simulink model "System_Design_Quadrocopter"  (Simulink 7.5)
settings: Solver=ode45  StartTime=0.0  StopTime=30  RelTol=1e-3
values from neighbouring files (symbols this model uses):
  phi0 = 0.15    [Quadrocopter_control_Driver.m]    (also in calc_stability.m = 0)
  r_phi0 = 0    [Quadrocopter_control_Driver.m]    (also in calc_stability.m)
  r_psi0 = 0    [Quadrocopter_control_Driver.m]    (also in calc_stability.m)
  r_theta0 = 0    [Quadrocopter_control_Driver.m]    (also in calc_stability.m)
  theta0 = 0.15    [Quadrocopter_control_Driver.m]    (also in calc_stability.m = 0)
  Ts = 0.01    [Reglerauslegung.m]    (also in Test_Reglerauslegung.m)
undefined symbols (not defined in the file or in its folder): bodyCtrl_phiCtrl_KD, bodyCtrl_phiCtrl_KI, bodyCtrl_phiCtrl_KP, bodyCtrl_rphiCtrl_KD, bodyCtrl_rphiCtrl_KI, bodyCtrl_rphiCtrl_KP, bodyCtrl_rpsiCtrl_KD, bodyCtrl_rpsiCtrl_KI, bodyCtrl_rpsiCtrl_KP, bodyCtrl_rthetaCtrl_KD, bodyCtrl_rthetaCtrl_KI, bodyCtrl_rthetaCtrl_KP, bodyCtrl_thetaCtrl_KD, bodyCtrl_thetaCtrl_KI, bodyCtrl_thetaCtrl_KP, boom, f1, f2, f3, f4, f5, g, I_x, I_y, I_z, m, positionCtrl_rpsiCtrl_KD, positionCtrl_rpsiCtrl_KI, positionCtrl_rpsiCtrl_KP, sigbuilder_block, speed, thrust, Ts_Opt
libraries: simulink x39, dspobslib x4, Copter_Library x3, Control_lib x1, sdolib x1
(part 4 of 4)

== stateflow chart Quadrocopter/Control/PID_Control_IMU only Trans (OC)/Hover Mode Enable ==
  state Hovering
    Control=1;
  state NotHovering
    Control=0;
  state WaitForBodyCtrl
    Control=0;
  NotHovering -> WaitForBodyCtrl : [((thetaSet>-set_val_th) && (thetaSet<set_val_th)) && ((phiSet>-set_val_th) && (phiSet<set_val_th)) && ((r_psiSet>-set_val_th) && (r_psiSet<set_val_th))]
  WaitForBodyCtrl -> NotHovering [order 2] : [((phiSet<=-set_val_th) || (phiSet>=set_val_th)) || ((thetaSet<=-set_val_th) || (thetaSet>=set_val_th)) || ((r_psiSet<=-set_val_th) || (r_psiSet>=set_val_th))]
  (default) -> NotHovering
  Hovering -> NotHovering : [((phiSet<=-set_val_th) || (phiSet>=set_val_th)) || ((thetaSet<=-set_val_th) || (thetaSet>=set_val_th)) || ((r_psiSet<=-set_val_th) || (r_psiSet>=set_val_th))]
  WaitForBodyCtrl -> Hovering [order 1] : after(1,sec)
  data: Control output double; phiSet input double; thetaSet input double; r_psiSet input double; set_val_th input double

== matlab function Quadrocopter/Sensors/Optical System/Rotation rpsi/Embedded MATLAB Function ==
  data: Sig input double; Fac output double; Gain input double
function Fac = fcn(Sig, Gain)
%#eml

Fac=Sig/Gain;

== matlab function Quadrocopter/Sensors/Optical System/Translation VX/Embedded MATLAB Function ==
  data: Sig input double; Fac output double; Gain input double
function Fac = fcn(Sig, Gain)
%#eml

Fac=Sig/Gain;

== matlab function Quadrocopter/Sensors/Optical System/Translation VY/Embedded MATLAB Function ==
  data: Sig input double; Fac output double; Gain input double
function Fac = fcn(Sig, Gain)
%#eml

Fac=Sig/Gain;

== matlab function Quadrocopter/Sim Ctrl/Embedded MATLAB Function ==
  data: ErrorGains input double; threshold output double; perCent input double
function threshold = fcn(ErrorGains, perCent)
%#eml
threshold=0;
if(ErrorGains(1) > 0 || ErrorGains(2) > 0 || ErrorGains(3) > 0 || ErrorGains(4) > 0)
   threshold = max(ErrorGains)*perCent;
end

== matlab function Quadrocopter/Sim Ctrl/Embedded MATLAB Function1 ==
  data: ErrorGains input double; u input double; ret output double
function ret = checkSimEnd(ErrorGains,u)
%#eml
persistent cnt1;
persistent cnt2;
persistent cnt3;
persistent first_time;
persistent lim;

if isempty(first_time)
first_time=1;
cnt1=0;
cnt2=0;
cnt3=0;
lim=50000;
end
ret=0;

if(ErrorGains(1) > 0 || ErrorGains(2) > 0 || ErrorGains(3) > 0 || ErrorGains(4) > 0)

    if(u(2) < abs(u(1)) && u(2) > -abs(u(1)))
      cnt1=cnt1+1;
    else
       cnt1=0; 
    end
    if(u(3) < abs(u(1)) && u(3) > -abs(u(1)))
     cnt2=cnt2+1;
    else
     cnt2=0;    
    end
    if(u(4) < abs(u(1)) && u(4) > -abs(u(1)))
      cnt3=cnt3+1;
    else
       cnt3=0; 
    end
    if(cnt1 > lim && cnt2 > lim && cnt3 > lim)
        ret=1;
    else
        ret=0;
    end
end

== stateflow chart Quadrocopter/Control/PID_Control_IMU Rot Trans (OC)/Hover Mode Enable ==
  state Hovering
    Control=1;
  state NotHovering
    Control=0;
  state WaitForBodyCtrl
    Control=0;
  NotHovering -> WaitForBodyCtrl : [((thetaSet>-set_val_th) && (thetaSet<set_val_th)) && ((phiSet>-set_val_th) && (phiSet<set_val_th)) && ((r_psiSet>-set_val_th) && (r_psiSet<set_val_th))]
  WaitForBodyCtrl -> NotHovering [order 2] : [((phiSet<=-set_val_th) || (phiSet>=set_val_th)) || ((thetaSet<=-set_val_th) || (thetaSet>=set_val_th)) || ((r_psiSet<=-set_val_th) || (r_psiSet>=set_val_th))]
  (default) -> NotHovering
  Hovering -> NotHovering : [((phiSet<=-set_val_th) || (phiSet>=set_val_th)) || ((thetaSet<=-set_val_th) || (thetaSet>=set_val_th)) || ((r_psiSet<=-set_val_th) || (r_psiSet>=set_val_th))]
  WaitForBodyCtrl -> Hovering [order 1] : after(1,sec)
  data: Control output double; phiSet input double; thetaSet input double; r_psiSet input double; set_val_th input double

== stateflow chart Quadrocopter/Control/PID_Control_IMU Rot Trans (OC) EMP/Hover Mode Enable ==
  state Hovering
    Control=1;
  state NotHovering
    Control=0;
  state WaitForBodyCtrl
    Control=0;
  NotHovering -> WaitForBodyCtrl : [((thetaSet>-set_val_th) && (thetaSet<set_val_th)) && ((phiSet>-set_val_th) && (phiSet<set_val_th)) && ((r_psiSet>-set_val_th) && (r_psiSet<set_val_th))]
  WaitForBodyCtrl -> NotHovering [order 2] : [((phiSet<=-set_val_th) || (phiSet>=set_val_th)) || ((thetaSet<=-set_val_th) || (thetaSet>=set_val_th)) || ((r_psiSet<=-set_val_th) || (r_psiSet>=set_val_th))]
  (default) -> NotHovering
  Hovering -> NotHovering : [((phiSet<=-set_val_th) || (phiSet>=set_val_th)) || ((thetaSet<=-set_val_th) || (thetaSet>=set_val_th)) || ((r_psiSet<=-set_val_th) || (r_psiSet>=set_val_th))]
  WaitForBodyCtrl -> Hovering [order 1] : after(1,sec)
  data: Control output double; phiSet input double; thetaSet input double; r_psiSet input double; set_val_th input double
